simulink model "SimpleLQR"  (R2020b)
settings: Solver=VariableStepDiscrete  StartTime=0.0  StopTime=100  MaxStep=0.01  RelTol=1e-3
values from neighbouring files (symbols this model uses):
  L = 0.189    [NonlinearVehicleLQR.m]    (also in NonlinearVehicleiLQR.m; linearVehicleiLQR.m)
  Q = [1 0 0; 0 1 0; 0 0 10]    [LQR.m]    (also in NonlinearVehicleLQR.m = eye(3)*10; NonlinearVehicleiLQR.m = eye(3)*10; SringiLQR.m = [1 0; 0 1]*1; SringiLQR2.m = [1 0; 0 1]*1)
  Qf = eye(3)    [LQR.m]    (also in NonlinearVehicleLQR.m; NonlinearVehicleiLQR.m; SringiLQR.m = [1 0; 0 1]; SringiLQR2.m = [1 0; 0 1])
  R = eye(2)*10^-4    [LQR.m]    (also in NonlinearVehicleLQR.m = eye(2)*10^-2; NonlinearVehicleiLQR.m = eye(2)*10^-2; SringiLQR.m = eye(1)*1e-2; SringiLQR2.m = eye(1)*1e-2)
  Radius = 0.02    [NonlinearVehicleLQR.m]    (also in NonlinearVehicleiLQR.m; linearVehicleiLQR.m)
undefined symbols (not defined in the file or in its folder): DiscIntNeverNeededParam
libraries: simulink x1
settings Model: Creator=iris  LastModifiedBy=iris

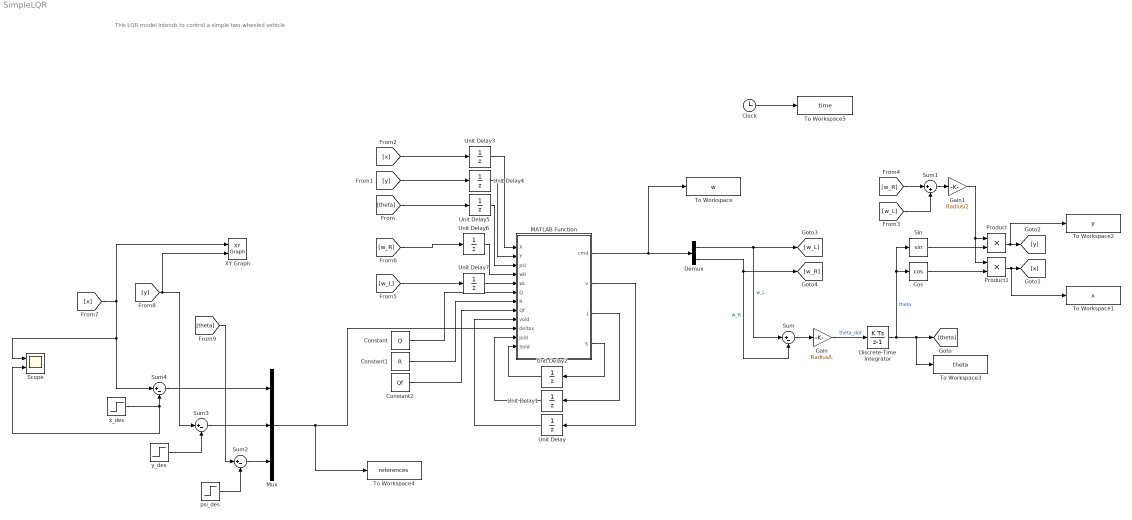
== system SimpleLQR ==
  note: This LQR model intends to control a simple two-wheeled vehicle
  Clock : Clock
  Constant : Constant  Value=Q
  Constant1 : Constant  Value=R
  Constant2 : Constant  Value=Qf
  Cos : Trigonometry  Operator=cos
  Demux : Demux  Outputs=2
  Discrete-Time Integrator : DiscreteIntegrator  SampleTime=-1  ICPrevOutput=DiscIntNeverNeededParam  ICPrevScaledInput=DiscIntNeverNeededParam
  Gain : Gain  Gain=Radius/L
  Gain1 : Gain  Gain=Radius/2
  MATLAB Function : MATLAB Function  TreatAsAtomicUnit=on
  Mux : Mux  Inputs=3
  Product : Product
  Product1 : Product
  Scope : Scope  NumInputPorts=2
  Sin : Trigonometry
  Sum{,2..4} (4 alike) : Sum  Inputs=|+-
  Sum1 : Sum  Inputs=|++
  To Workspace : ToWorkspace  VariableName=w  SampleTime=-1
  To Workspace1 : ToWorkspace  VariableName=x  SampleTime=-1
  To Workspace2 : ToWorkspace  VariableName=y  SampleTime=-1
  To Workspace3 : ToWorkspace  VariableName=theta  SampleTime=-1
  To Workspace4 : ToWorkspace  VariableName=references  SampleTime=-1
  To Workspace5 : ToWorkspace  VariableName=time  SampleTime=-1
  Unit Delay : UnitDelay  InitialCondition=zeros(3,1)  SampleTime=-1  HasFrameUpgradeWarning=on
  Unit Delay1 : UnitDelay  InitialCondition=1  SampleTime=-1  HasFrameUpgradeWarning=on
  Unit Delay2 : UnitDelay  InitialCondition=Qf  SampleTime=-1  HasFrameUpgradeWarning=on
  Unit Delay{3..7} (5 alike) : UnitDelay  SampleTime=-1  HasFrameUpgradeWarning=on
  XY Graph : simulink/Sinks/XY Graph  xmin=-5  xmax=5  ymin=-5  ymax=5  st=-1
  psi_des : Step  SampleTime=0
  x_des : Step  SampleTime=0
  y_des : Step  SampleTime=0
  wires:
  MATLAB Function/3(J) -> Unit Delay1/1
  Unit Delay1/1 -> MATLAB Function/11(Jold)
  MATLAB Function/4(S) -> Unit Delay2/1
  Unit Delay2/1 -> MATLAB Function/12(Sold)
  MATLAB Function/2(v) -> Unit Delay/1
  Unit Delay/1 -> MATLAB Function/9(vold)
  MATLAB Function/1(cmd) -> To Workspace/1, Demux/1
  Demux/1 -> Sum/1, [w_L]  "w_L"
  Demux/2 -> Sum/2, [w_R]  "w_R"
  Sum/1 -> Gain/1
  Gain/1 -> Discrete-Time Integrator/1  "theta_dot"
  Discrete-Time Integrator/1 -> Sin/1, Cos/1, To Workspace3/1, [theta]  "theta"
  [theta] -> Unit Delay5/1
  [x] -> Unit Delay3/1
  [y] -> Unit Delay4/1
  [w_R] -> Sum1/1
  [w_L] -> Sum1/2
  Cos/1 -> Product1/2
  Sin/1 -> Product/2
  Sum1/1 -> Gain1/1
  Gain1/1 -> Product1/1, Product/1
  Product1/1 -> To Workspace1/1, [x]
  Product/1 -> To Workspace2/1, [y]
  [w_L] -> Unit Delay7/1
  [w_R] -> Unit Delay6/1
  Constant/1 -> MATLAB Function/6(Q)
  Constant1/1 -> MATLAB Function/7(R)
  Constant2/1 -> MATLAB Function/8(Qf)
  Mux/1 -> To Workspace4/1, MATLAB Function/10(deltax)
  [theta] -> Sum2/1
  [x] -> Sum4/1, Scope/1, XY Graph/1
  y_des/1 -> Sum3/2
  Sum2/1 -> Mux/3
  Sum4/1 -> Mux/1
  Sum3/1 -> Mux/2
  psi_des/1 -> Sum2/2
  x_des/1 -> Scope/2, Sum4/2
  Unit Delay3/1 -> MATLAB Function/1(X)
  Unit Delay4/1 -> MATLAB Function/2(Y)
  Unit Delay5/1 -> MATLAB Function/3(psi)
  Unit Delay6/1 -> MATLAB Function/4(wR)
  Unit Delay7/1 -> MATLAB Function/5(wL)
  Clock/1 -> To Workspace5/1
  [y] -> XY Graph/2, Sum3/1

== matlab function SimpleLQR/MATLAB Function ==
  data: X input; cmd output; Y input; psi input; wR input; wL input; Q input; R input; Qf input; vold input; deltax input; Jold input; Sold input; v output; J output; S output
function [cmd, v, J, S]= fcn(X, Y, psi, wR, wL, Q, R, Qf, vold, deltax, Jold, Sold)

r = 0.02;
B = 0.185;
dt = 0.01;

toll = 3*10^-5;

A = [1 0 dt*-sin(psi)*r/2*(wR+wL);...
     0 1 dt*cos(psi)*r/2*(wR+wL);...
     0 0 1];
B = dt*[cos(psi)*r/2 cos(psi)*r/2;...
     sin(psi)*r/2 sin(psi)*r/2;...
     -r/B r/B];

J = [X Y psi]*Qf*[X Y psi]'+[X Y psi]*Q*[X Y psi]'+[wL wR]*R*[wL wR]';

cmd = zeros(2,1);

if abs(Jold-J)/Jold > toll
    K  = (B'*Sold*B+R)\B'*Sold*A;
    Kv = (B'*Sold*B+R)\B';
    Ku = (B'*Sold*B+R)\R;
    S  = A'*Sold*(A-B*K)+Q;
    v  = (A-B*K)'*vold-K'*R*[wL wR]'+Q*[X Y psi]';

    deltau = -K*deltax-Kv*v-Ku*[wL wR]';
    cmd  = [wL wR]' + deltau;
else
    S  = Sold;
    v  = vold;
    cmd  = [wL wR]';
end
